simulink model "motorPulseFilt2"  (R2019b)
settings: Solver=ode4  StartTime=0.0  StopTime=5  FixedStep=Ts  RelTol=1e-3  EnableMultiTasking=on
values from neighbouring files (symbols this model uses):
  Ts = 8    [matlab.mat]
libraries: arduino_io_lib x6
settings Model: SILPILModeSetting=veronly  ExtModeTrigDuration=2  Creator=gcampa  LastModifiedBy=EK
settings DataIOCC: LimitDataPoints=on  SaveFormat=Array  SignalLoggingSaveFormat=ModelDataLogs  ReturnWorkspaceOutputs=off
settings OptimizationCC: EnhancedBackFolding=on  PassReuseOutputArgsAs=Individual arguments  ZeroExternalMemoryAtStartup=off  ZeroInternalMemoryAtStartup=off  MaxStackSize=64  OptimizeBlockOrder=speed  DifferentSizesBufferReuse=on  OptimizationCustomize=off  EfficientTunableParamExpr=on
settings DebuggingCC: UnderspecifiedInitializationDetection=Classic  MergeDetectMultiDrivingBlocksExec=none  MultiTaskDSMMsg=warning  MultiTaskCondExecSysMsg=none  ParameterTunabilityLossMsg=error  SFUnexpectedBacktrackingDiag=warning  SFNoUnconditionalDefaultTransitionDiag=warning  SFExecutionAtInitializationDiag=none  ArithmeticOperatorsInVariantConditions=warning
settings HardwareCC: ProdBitPerInt=16  ProdBitPerPointer=16  ProdBitPerSizeT=16  ProdBitPerPtrDiffT=16  ProdLargestAtomicFloat=None  ProdWordSize=8  ProdHWDeviceType=Atmel->AVR
settings ModelReferenceCC: PropagateSignalLabelsOutOfModel=off
settings SFSimCC: SimUseLocalCustomCode=off  MATLABDynamicMemAlloc=off  CustomCodeUndefinedFunction=UseInterfaceOnly
settings RTWCC: SystemTargetFile=ert.tlc  HardwareBoard=Arduino Uno  TLCOptions=-aInlineSetEventsForThisBaseRateFcn=TLC_FALSE -aSuppressMultiTaskScheduler=TLC_FALSE -aRateBasedStepFcn=1  TemplateMakefile=ert_default_tmf  GenerateReport=on  RTWVerbose=off  RTWUseLocalCustomCode=off  Toolchain=Arduino AVR  BuildConfiguration=Faster Runs  IncludeHyperlinkInReport=on  LaunchReport=on  GenerateTraceInfo=on  GenerateTraceReport=on  GenerateTraceReportSl=on  GenerateTraceReportSf=on  GenerateTraceReportEml=on
settings CodeAppCC: ForceParamTrailComments=on  IgnoreCustomStorageClasses=off  OperatorAnnotations=on  SimulinkDataObjDesc=on  SFDataObjDesc=on  InsertBlockDesc=on
settings ERTTargetCC: SupportContinuousTime=on  SupportVariableSizeSignals=on  ExtModeStaticAllocSize=250
settings ConfigComp: CovMetricSettings=dw  CovHtmlReporting=on  CovSaveCumulativeToWorkspaceVar=on  CovSaveSingleToWorkspaceVar=on  CovExternalEMLEnable=off

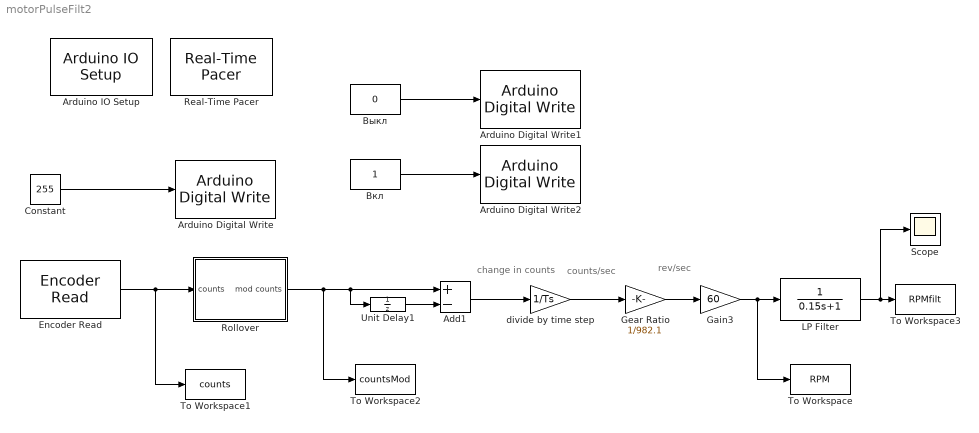
== system motorPulseFilt2 ==
  note: change
      | in counts
  note: rev/sec
  note: counts/sec
  Add1 : Sum  Inputs=+-
  Arduino Digital Write : arduino_io_lib/Arduino Digital Write  arduinoVar=Temporary arduino variable: Arduino1  arduinoPin=9  T=-1
      settings: SourceProductName=Arduino IO Library
  Arduino Digital Write1 : arduino_io_lib/Arduino Digital Write  arduinoVar=Temporary arduino variable: Arduino1  arduinoPin=4  T=0.2
      settings: SourceProductName=Arduino IO Library
  Arduino Digital Write2 : arduino_io_lib/Arduino Digital Write  arduinoVar=Temporary arduino variable: Arduino1  arduinoPin=5  T=0.2
      settings: SourceProductName=Arduino IO Library
  Arduino IO Setup : arduino_io_lib/Arduino IO Setup  Priority=3  arduinoVar=Temporary arduino variable: Arduino1  workspaceVarName=b  comPort=COM5
      settings: SourceProductName=Arduino IO Library
  Constant : Constant  Value=255
  Encoder Read : arduino_io_lib/Encoder Read  arduinoVar=Temporary arduino variable: Arduino1  encNum=1  pinA=2  pinB=3  DbDl=0  T=Ts
      settings: SourceProductName=Arduino IO Library
  Gain3 : Gain  Gain=60
  Gear Ratio : Gain  Gain=1/982.1
  LP Filter : TransferFcn  Denominator=[0.15 1]
  Real-Time Pacer : arduino_io_lib/Real-Time Pacer  simTimePerRealTime=1
      settings: SourceProductName=Arduino IO Library
  Rollover : Subsystem
  Scope : Scope
  To Workspace : ToWorkspace  VariableName=RPM  SaveFormat=Timeseries  SampleTime=-1
  To Workspace1 : ToWorkspace  VariableName=counts  SaveFormat=Timeseries  SampleTime=-1
  To Workspace2 : ToWorkspace  VariableName=countsMod  SaveFormat=Timeseries  SampleTime=-1
  To Workspace3 : ToWorkspace  VariableName=RPMfilt  SaveFormat=Timeseries  SampleTime=-1
  Unit Delay1 : UnitDelay  SampleTime=-1  HasFrameUpgradeWarning=on
  divide by time step : Gain  Gain=1/Ts
  Вкл : Constant  SampleTime=-1
  Выкл : Constant  Value=0  SampleTime=-1
  wires:
  Unit Delay1/1 -> Add1/2
  Gear Ratio/1 -> Gain3/1
  Gain3/1 -> LP Filter/1, To Workspace/1
  Constant/1 -> Arduino Digital Write/1
  divide by time step/1 -> Gear Ratio/1
  Add1/1 -> divide by time step/1
  LP Filter/1 -> Scope/1, To Workspace3/1
  Rollover/1(" mod counts") -> To Workspace2/1, Add1/1, Unit Delay1/1
  Encoder Read/1 -> To Workspace1/1, Rollover/1(counts)
  Вкл/1 -> Arduino Digital Write2/1
  Выкл/1 -> Arduino Digital Write1/1

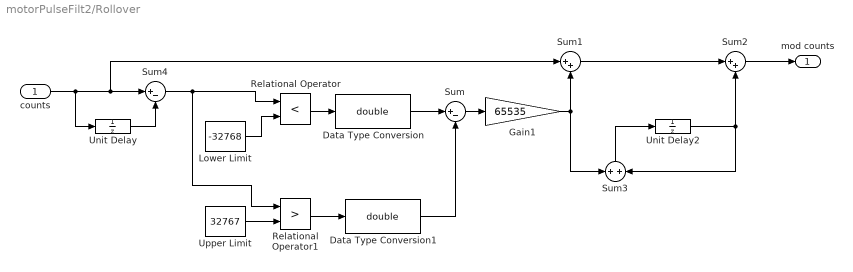
== system motorPulseFilt2/Rollover ==
  counts : Inport
  " Lower Limit" : Constant  Value=-32768
  " Upper Limit" : Constant  Value=32767
  Data Type Conversion : DataTypeConversion  OutDataTypeStr=double  RndMeth=Zero
  Data Type Conversion1 : DataTypeConversion  OutDataTypeStr=double  RndMeth=Zero
  Gain1 : Gain  Gain=65535
  Relational Operator : RelationalOperator  Operator=<  OutDataTypeStr=boolean  RndMeth=Nearest
  Relational Operator1 : RelationalOperator  Operator=>  OutDataTypeStr=boolean  RndMeth=Nearest
  Sum : Sum  Inputs=|+-
  Sum1 : Sum  Inputs=|++
  Sum2 : Sum  Inputs=|++
  Sum3 : Sum
  Sum4 : Sum  Inputs=|+-
  Unit Delay : UnitDelay  SampleTime=-1  HasFrameUpgradeWarning=on
  Unit Delay2 : UnitDelay  SampleTime=-1  HasFrameUpgradeWarning=on
  " mod counts" : Outport
  wires:
  counts/1 -> Unit Delay/1, Sum1/1, Sum4/1
  Sum2/1 -> " mod counts"/1
  Unit Delay/1 -> Sum4/2
  Data Type Conversion/1 -> Sum/1
  Sum3/1 -> Unit Delay2/1
  Data Type Conversion1/1 -> Sum/2
  Sum/1 -> Gain1/1
  Gain1/1 -> Sum1/2, Sum3/1
  Relational Operator1/1 -> Data Type Conversion1/1
  Sum1/1 -> Sum2/1
  Relational Operator/1 -> Data Type Conversion/1
  " Upper Limit"/1 -> Relational Operator1/2
  Unit Delay2/1 -> Sum3/2, Sum2/2
  " Lower Limit"/1 -> Relational Operator/2
  Sum4/1 -> Relational Operator/1, Relational Operator1/1
